simulink model "fk_ee"  (R2020a)
settings: Solver=VariableStepAuto  StartTime=0.0  StopTime=10.0  RelTol=1e-3
libraries: simulink x3, dsppolyfun x2
settings Model: Creator=UNIST  LastModifiedBy=UNIST

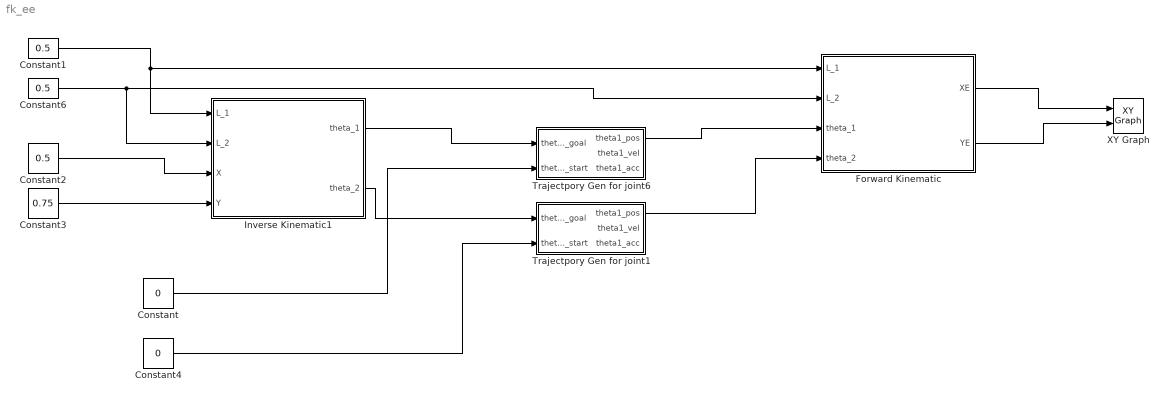
== system fk_ee ==
  Constant : Constant  Value=0
  Constant1 : Constant  Value=0.5
  Constant2 : Constant  Value=0.5
  Constant3 : Constant  Value=0.75
  Constant4 : Constant  Value=0
  Constant6 : Constant  Value=0.5
  Forward Kinematic : MATLAB Function  TreatAsAtomicUnit=on
  Inverse Kinematic1 : MATLAB Function  TreatAsAtomicUnit=on
  Trajectpory Gen for joint1 : Subsystem
  Trajectpory Gen for joint6 : Subsystem
  XY Graph : simulink/Sinks/XY Graph  xmin=-1  xmax=1  ymin=-1  ymax=1  st=-1
  wires:
  Constant2/1 -> Inverse Kinematic1/3(X)
  Constant3/1 -> Inverse Kinematic1/4(Y)
  Constant6/1 -> Inverse Kinematic1/2(L_2), Forward Kinematic/2(L_2)
  Constant1/1 -> Inverse Kinematic1/1(L_1), Forward Kinematic/1(L_1)
  Inverse Kinematic1/1(theta_1) -> Trajectpory Gen for joint6/1("theta1_goal ")
  Constant4/1 -> Trajectpory Gen for joint1/2("theta1_start ")
  Inverse Kinematic1/2(theta_2) -> Trajectpory Gen for joint1/1("theta1_goal ")
  Constant/1 -> Trajectpory Gen for joint6/2("theta1_start ")
  Trajectpory Gen for joint6/1("theta1_pos ") -> Forward Kinematic/3(theta_1)
  Trajectpory Gen for joint1/1("theta1_pos ") -> Forward Kinematic/4(theta_2)
  Forward Kinematic/1(XE) -> XY Graph/1
  Forward Kinematic/2(YE) -> XY Graph/2

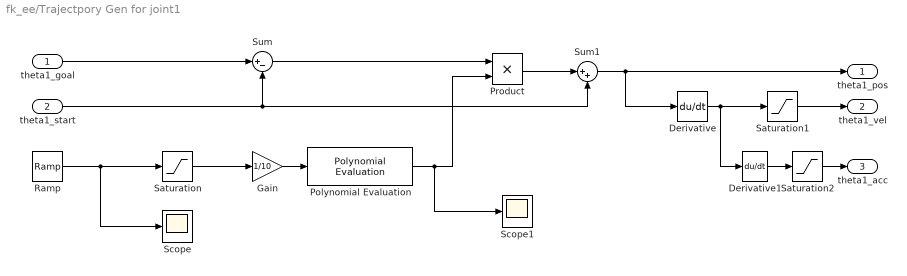
== system fk_ee/Trajectpory Gen for joint1 ==
  "theta1_goal " : Inport
  "theta1_start " : Inport  Port=2
  Derivative : Derivative
  Derivative1 : Derivative
  Gain : Gain  Gain=1/10
  Polynomial Evaluation : dsppolyfun/Polynomial Evaluation  useConstCoeffs=on  constCoeffs=[6 -15 10 0 0 0]
      settings: SourceProductBaseCode=DS
  Product : Product
  Ramp : simulink/Sources/Ramp  slope=1  start=0  InitialOutput=0
  Saturation : Saturate  UpperLimit=10  LowerLimit=-10
  Saturation1 : Saturate
  Saturation2 : Saturate
  Scope : Scope
  Scope1 : Scope
  Sum : Sum  Inputs=|+-
  Sum1 : Sum  Inputs=|++
  "theta1_pos " : Outport  VectorParamsAs1DForOutWhenUnconnected=off
  "theta1_vel " : Outport  Port=2  VectorParamsAs1DForOutWhenUnconnected=off
  "theta1_acc " : Outport  Port=3  VectorParamsAs1DForOutWhenUnconnected=off
  wires:
  "theta1_start "/1 -> Sum1/2, Sum/2
  Sum/1 -> Product/1
  "theta1_goal "/1 -> Sum/1
  Sum1/1 -> Derivative/1, "theta1_pos "/1
  Derivative1/1 -> Saturation2/1
  Saturation1/1 -> "theta1_vel "/1
  Gain/1 -> Polynomial Evaluation/1
  Product/1 -> Sum1/1
  Polynomial Evaluation/1 -> Scope1/1, Product/2
  Saturation2/1 -> "theta1_acc "/1
  Saturation/1 -> Gain/1
  Derivative/1 -> Derivative1/1, Saturation1/1
  Ramp/1 -> Scope/1, Saturation/1

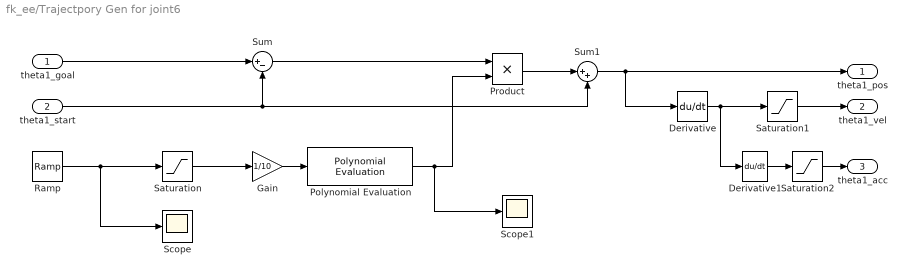
== system fk_ee/Trajectpory Gen for joint6 ==
  "theta1_goal " : Inport
  "theta1_start " : Inport  Port=2
  Derivative : Derivative
  Derivative1 : Derivative
  Gain : Gain  Gain=1/10
  Polynomial Evaluation : dsppolyfun/Polynomial Evaluation  useConstCoeffs=on  constCoeffs=[6 -15 10 0 0 0]
      settings: SourceProductBaseCode=DS
  Product : Product
  Ramp : simulink/Sources/Ramp  slope=1  start=0  InitialOutput=0
  Saturation : Saturate  UpperLimit=10  LowerLimit=-10
  Saturation1 : Saturate
  Saturation2 : Saturate
  Scope : Scope
  Scope1 : Scope
  Sum : Sum  Inputs=|+-
  Sum1 : Sum  Inputs=|++
  "theta1_pos " : Outport  VectorParamsAs1DForOutWhenUnconnected=off
  "theta1_vel " : Outport  Port=2  VectorParamsAs1DForOutWhenUnconnected=off
  "theta1_acc " : Outport  Port=3  VectorParamsAs1DForOutWhenUnconnected=off
  wires:
  "theta1_start "/1 -> Sum1/2, Sum/2
  Sum/1 -> Product/1
  "theta1_goal "/1 -> Sum/1
  Sum1/1 -> Derivative/1, "theta1_pos "/1
  Derivative1/1 -> Saturation2/1
  Saturation1/1 -> "theta1_vel "/1
  Gain/1 -> Polynomial Evaluation/1
  Product/1 -> Sum1/1
  Polynomial Evaluation/1 -> Scope1/1, Product/2
  Saturation2/1 -> "theta1_acc "/1
  Saturation/1 -> Gain/1
  Derivative/1 -> Derivative1/1, Saturation1/1
  Ramp/1 -> Scope/1, Saturation/1

== matlab function fk_ee/Inverse Kinematic1 ==
  data: L_1 input; L_2 input; theta_1 output; X input; Y input; theta_2 output
function [theta_1,theta_2] = IK_2(L_1, L_2, X,Y)
temp = (X^2+Y^2-L_1^2-L_2^2)/(2*L_1*L_2);
k =sqrt(1-temp^2);
theta_2 = atan2(k,temp);

theta_1 = atan2(Y,X)-atan2(L_2*sin(theta_2),L_1+L_2*cos(theta_2));
end

== matlab function fk_ee/Forward Kinematic ==
  data: L_1 input; XE output; L_2 input; theta_1 input; theta_2 input; YE output
function [XE,YE] = THE_XEYE(L_1,L_2,theta_1,theta_2)
theta_1 = rad2deg(theta_1);
theta_2 = rad2deg(theta_2);
XE = L_2.*cos(theta_1+theta_2)+L_1.*cos(theta_1);
if nargout > 1
    YE = L_2.*sin(theta_1+theta_2)+L_1.*sin(theta_1);
end
